simulink model "Perfect_Lineaer"  (R2017a)
settings: Solver=VariableStepAuto  StartTime=0.0  StopTime=17  FixedStep=0.01  RelTol=1e-3
values from neighbouring files (symbols this model uses):
  A = [-4.65E-06	0.0001701	-0.0002836	0	0	0	-2.56E-06	-7.97E-06	3.61E-06 ... (first row only)    [surfaces_setup_test.m]
  A0 = [-4.65E-06	0.0001701	-0.0002836	0	0	0	0	-1.43	0 ... (first row only)    [surfaces_setup_test.m]
  a0_s2345 = [0;0;0.05;0.05]    [HW5_4_surfaces.m]    (also in TEST_aerosetup.m; surfaces_setup_test.m)
  A_2345 = c_2345.*b_2345    [HW5_4_surfaces.m]    (also in TEST_aerosetup.m; surfaces_setup_test.m)
  Aileron_left = 0    [HW5_4_surfaces.m]    (also in TEST_aerosetup.m; surfaces_setup_test.m)
  Aileron_right = 0    [HW5_4_surfaces.m]    (also in TEST_aerosetup.m; surfaces_setup_test.m)
  B = [-7.98E-09	7.83E-09	1.68E-09	2.75E-10 ... (first row only)    [surfaces_setup_test.m]
  B0 = [-6.2	6.2	0	0.45 ... (first row only)    [surfaces_setup_test.m]
  c_2345 = [0.075;0.08;0.1;0.1]    [HW5_4_surfaces.m]    (also in TEST_aerosetup.m; surfaces_setup_test.m)
  CD0_s2345 = [0.01;0.01;0.01;0.01]    [HW5_4_surfaces.m]    (also in TEST_aerosetup.m; surfaces_setup_test.m)
  CDa_s2345 = [1;1;1;1]    [HW5_4_surfaces.m]    (also in TEST_aerosetup.m; surfaces_setup_test.m)
  CL0_2345 = [0;0; 0.05; 0.05]    [HW5_4_surfaces.m]    (also in TEST_aerosetup.m; surfaces_setup_test.m)
  CLa = 2*pi*(r./(2+r))    [HW5_4_surfaces.m]    (also in TEST_aerosetup.m; surfaces_setup_test.m)
  CM0_s2345 = [0;0;-0.05;-0.05]    [HW5_4_surfaces.m]    (also in TEST_aerosetup.m; surfaces_setup_test.m)
  CMa_s2345 = [0; 0; 0; 0]    [HW5_4_surfaces.m]    (also in TEST_aerosetup.m; surfaces_setup_test.m)
  e_s2345 = [0.8;0.8;0.9;0.9]    [HW5_4_surfaces.m]    (also in TEST_aerosetup.m; surfaces_setup_test.m)
  elevator = 0    [HW5_4_surfaces.m]    (also in TEST_aerosetup.m; surfaces_setup_test.m)
  Fext_N = -g_EN * m    [HW5_4_surfaces.m]    (also in TEST_aerosetup.m = [10 10 10]; surfaces_setup_test.m)
  g_EN = [0; 0; 9.81]    [HW5_4_surfaces.m]    (also in TEST_aerosetup.m = [0; 0; 9.8]; surfaces_setup_test.m)
  i_s2345 = [0; 0; 0.05; 0.05;]    [HW5_4_surfaces.m]    (also in TEST_aerosetup.m; surfaces_setup_test.m)
  J_cgp = ones(3)    [surfaces_setup_test.m]
  M_total = sum(MnG(:,1))/1000    [HW5_4_surfaces.m]    (also in TEST_aerosetup.m; surfaces_setup_test.m = sum(MnG1(:,1))/1000)
  Mext_B = [0; 0; 0]    [HW5_4_surfaces.m]    (also in TEST_aerosetup.m = [1; 1; 1]; surfaces_setup_test.m)
  p_E_BE_ini = p_E_BE_ini_deg .* [deg2rad; deg2rad; 1]    [HW5_4_surfaces.m]    (also in TEST_aerosetup.m; surfaces_setup_test.m)
  r = b_2345./c_2345    [HW5_4_surfaces.m]    (also in TEST_aerosetup.m; surfaces_setup_test.m)
  Rearth = 6371000    [HW5_4_surfaces.m]    (also in TEST_aerosetup.m; surfaces_setup_test.m)
  rudder = 0    [HW5_4_surfaces.m]    (also in TEST_aerosetup.m; surfaces_setup_test.m)
  Theta_ini = Theta_ini_deg * deg2rad    [HW5_4_surfaces.m]    (also in TEST_aerosetup.m; surfaces_setup_test.m)
  U0 = [Aileron_right;Aileron_left;elevator;rudder]    [surfaces_setup_test.m]
  v_N_AE = [0;0;0]    [HW5_4_surfaces.m]    (also in TEST_aerosetup.m; surfaces_setup_test.m)
  Vbbe_int = [10; 0; 0]    [HW5_4_surfaces.m]    (also in TEST_aerosetup.m; surfaces_setup_test.m = [5; 0; 0])
  w_B_BE_ini = [1e0; 1e-2; 1e-2]    [HW5_4_surfaces.m]    (also in TEST_aerosetup.m; surfaces_setup_test.m)
  X0 = [w_B_BE_ini;Theta_ini;Vbbe_int]    [surfaces_setup_test.m]
  xyz_s = [[-0.76 0 0.16];[-0.76 0 -0.09];[-0.23 0.44 0];[-0.23 -0.44 0];]    [HW5_4_surfaces.m]    (also in TEST_aerosetup.m; surfaces_setup_test.m)
undefined symbols (not defined in the file or in its folder): Discrete, Earth, K, Time, WGS84
libraries: simulink x83, aerolibfltsims x5, dspsrcs4 x4, simulink_extras x4, dspinverses x3, vrlib x2, sharedtransform x1, aerolibtransform2 x1, aerolibutil x1, sharedutil x1, ctrlSharedLib x1
(part 6 of 8)

== system Perfect_Lineaer/Skid to turn (Lateral Dynamics)1/Subsystem3 ==
  note: Inner loop
  note: State loop
  Rudder : Inport
  A : Gain  Gain=A  Multiplication=Matrix(K*u)
  B : Gain  Gain=B  Multiplication=Matrix(K*u)
  Constant1 : Constant  Value=0
  Constant2 : Constant  Value=X0
  Demux : Demux  Outputs=9
  Integrator : Integrator  InitialConditionSource=external
  KD_Based on Rlocus : Gain
  Mux : Mux  Inputs=9
  Mux1 : Mux
  Scope : Scope
  Scope1 : Scope
  Sum : Sum  Inputs=|++
  Sum1 : Sum  Inputs=|++
  Sum4 : Sum  Inputs=|+-
  selector : Subsystem
  R(yaw) : Outport
  wires:
  Demux/7 -> Mux/7
  Demux/6 -> Mux/6
  Constant2/1 -> Integrator/2
  Demux/3 -> Mux/3
  Sum/1 -> Integrator/1
  selector/1(Out1) -> Scope1/1, KD_Based on Rlocus/1
  B/1 -> Demux/1
  Demux/2 -> Mux/2
  Demux/4 -> Mux/4
  Demux/9 -> Mux/9
  Integrator/1 -> selector/1(In1), Sum4/2, Scope/1, A/1
  Sum4/1 -> Sum/1
  A/1 -> Sum/2
  Demux/5 -> Mux/5
  Demux/1 -> Mux/1
  Mux/1 -> Sum4/1
  Mux1/1 -> B/1
  Constant1/1 -> Mux1/3, Mux1/2, Mux1/1
  Rudder/1 -> Mux1/4
  selector/2(Out2) -> R(yaw)/1
  Demux/8 -> Sum1/1
  KD_Based on Rlocus/1 -> Sum1/2
  Sum1/1 -> Mux/8

== system Perfect_Lineaer/Skid to turn (Lateral Dynamics)1/Subsystem4 ==
  note: Inner loop
  note: State loop
  Rudder : Inport
  A : Gain  Gain=A  Multiplication=Matrix(K*u)
  B : Gain  Gain=B  Multiplication=Matrix(K*u)
  Constant1 : Constant  Value=0
  Constant2 : Constant  Value=X0
  Demux : Demux  Outputs=9
  Integrator : Integrator  InitialConditionSource=external
  KD_Based on Rlocus : Gain
  Mux : Mux  Inputs=9
  Mux1 : Mux
  Scope : Scope
  Scope1 : Scope
  Sum : Sum  Inputs=|++
  Sum1 : Sum  Inputs=|++
  Sum4 : Sum  Inputs=|+-
  selector : Subsystem
  R(yaw) : Outport
  wires:
  Demux/7 -> Mux/7
  Demux/6 -> Mux/6
  Constant2/1 -> Integrator/2
  Demux/3 -> Mux/3
  Sum/1 -> Integrator/1
  selector/1(Out1) -> Scope1/1, KD_Based on Rlocus/1
  B/1 -> Demux/1
  Demux/2 -> Mux/2
  Demux/4 -> Mux/4
  Demux/9 -> Mux/9
  Integrator/1 -> selector/1(In1), Sum4/2, Scope/1, A/1
  Sum4/1 -> Sum/1
  A/1 -> Sum/2
  Demux/5 -> Mux/5
  Demux/1 -> Mux/1
  Mux/1 -> Sum4/1
  Mux1/1 -> B/1
  Constant1/1 -> Mux1/3, Mux1/2, Mux1/1
  Rudder/1 -> Mux1/4
  selector/2(Out2) -> R(yaw)/1
  Demux/8 -> Sum1/1
  KD_Based on Rlocus/1 -> Sum1/2
  Sum1/1 -> Mux/8

== system Perfect_Lineaer/Skid to turn (Lateral Dynamics)1/Subsystem5 ==
  note: Inner loop
  note: State loop
  Rudder : Inport
  Elevator : Inport  Port=2
  A : Gain  Gain=A  Multiplication=Matrix(K*u)
  B : Gain  Gain=B  Multiplication=Matrix(K*u)
  Constant1 : Constant  Value=0
  Constant2 : Constant  Value=X0
  Demux : Demux  Outputs=9
  Integrator : Integrator  InitialConditionSource=external
  KD_Based on Rlocus : Gain
  Mux : Mux  Inputs=9
  Mux1 : Mux
  Scope : Scope
  Scope1 : Scope
  Sum : Sum  Inputs=|++
  Sum1 : Sum  Inputs=|++
  Sum4 : Sum  Inputs=|+-
  selector : Subsystem
  R(yaw) : Outport
  Q(pitch) : Outport  Port=2
  wires:
  Demux/7 -> Mux/7
  Demux/6 -> Mux/6
  Constant2/1 -> Integrator/2
  Demux/3 -> Mux/3
  Sum/1 -> Integrator/1
  selector/1(Out1) -> Scope1/1, KD_Based on Rlocus/1
  B/1 -> Demux/1
  Demux/2 -> Mux/2
  Demux/4 -> Mux/4
  Demux/9 -> Mux/9
  Integrator/1 -> selector/1(In1), Sum4/2, Scope/1, A/1
  Sum4/1 -> Sum/1
  A/1 -> Sum/2
  Demux/5 -> Mux/5
  Demux/1 -> Mux/1
  Mux/1 -> Sum4/1
  Mux1/1 -> B/1
  Constant1/1 -> Mux1/2, Mux1/1
  Rudder/1 -> Mux1/4
  selector/2(yaw) -> R(yaw)/1
  Demux/8 -> Sum1/1
  KD_Based on Rlocus/1 -> Sum1/2
  Sum1/1 -> Mux/8
  selector/3(pitch) -> Q(pitch)/1
  Elevator/1 -> Mux1/3

== system Perfect_Lineaer/Skid to turn (Lateral Dynamics)1/Subsystem6 ==
  note: Inner loop
  note: State loop
  Rudder : Inport
  A : Gain  Gain=A  Multiplication=Matrix(K*u)
  B : Gain  Gain=B  Multiplication=Matrix(K*u)
  Constant1 : Constant  Value=0
  Constant2 : Constant  Value=X0
  Demux : Demux  Outputs=9
  Integrator : Integrator  InitialConditionSource=external
  KD_Based on Rlocus : Gain
  Mux : Mux  Inputs=9
  Mux1 : Mux
  Scope : Scope
  Scope1 : Scope
  Sum : Sum  Inputs=|++
  Sum1 : Sum  Inputs=|++
  Sum4 : Sum  Inputs=|+-
  selector : Subsystem
  R(yaw) : Outport
  wires:
  Demux/7 -> Mux/7
  Demux/6 -> Mux/6
  Constant2/1 -> Integrator/2
  Demux/3 -> Mux/3
  Sum/1 -> Integrator/1
  selector/1(Out1) -> Scope1/1, KD_Based on Rlocus/1
  B/1 -> Demux/1
  Demux/2 -> Mux/2
  Demux/4 -> Mux/4
  Demux/9 -> Mux/9
  Integrator/1 -> selector/1(In1), Sum4/2, Scope/1, A/1
  Sum4/1 -> Sum/1
  A/1 -> Sum/2
  Demux/5 -> Mux/5
  Demux/1 -> Mux/1
  Mux/1 -> Sum4/1
  Mux1/1 -> B/1
  Constant1/1 -> Mux1/3, Mux1/2, Mux1/1
  Rudder/1 -> Mux1/4
  selector/2(Out2) -> R(yaw)/1
  Demux/8 -> Sum1/1
  KD_Based on Rlocus/1 -> Sum1/2
  Sum1/1 -> Mux/8

== system Perfect_Lineaer/Skid to turn (Lateral Dynamics)1/Subsystem7 ==
  note: Inner loop
  note: State loop
  Aileron_r : Inport
  Aileron_l : Inport  Port=2
  A : Gain  Gain=A  Multiplication=Matrix(K*u)
  B : Gain  Gain=B  Multiplication=Matrix(K*u)
  Constant1 : Constant  Value=0
  Constant2 : Constant  Value=X0
  Demux : Demux  Outputs=9
  Integrator : Integrator  InitialConditionSource=external
  KD_Based on Rlocus : Gain
  Mux : Mux  Inputs=9
  Mux1 : Mux
  Scope : Scope
  Scope1 : Scope
  Sum : Sum  Inputs=|++
  Sum1 : Sum  Inputs=|++
  Sum4 : Sum  Inputs=|+-
  selector : Subsystem
  P(roll) : Outport
  wires:
  Demux/7 -> Mux/7
  Demux/6 -> Mux/6
  Constant2/1 -> Integrator/2
  Demux/3 -> Mux/3
  Sum/1 -> Integrator/1
  selector/1(Out1) -> Scope1/1, KD_Based on Rlocus/1
  B/1 -> Demux/1
  Demux/2 -> Mux/2
  Demux/4 -> Mux/4
  Demux/9 -> Mux/9
  Integrator/1 -> selector/1(In1), Sum4/2, Scope/1, A/1
  Sum4/1 -> Sum/1
  A/1 -> Sum/2
  Demux/5 -> Mux/5
  Demux/1 -> Mux/1
  Mux/1 -> Sum4/1
  Mux1/1 -> B/1
  Constant1/1 -> Mux1/3, Mux1/4
  selector/2(Out2) -> P(roll)/1
  Demux/8 -> Sum1/1
  KD_Based on Rlocus/1 -> Sum1/2
  Sum1/1 -> Mux/8
  Aileron_r/1 -> Mux1/1
  Aileron_l/1 -> Mux1/2

== system Perfect_Lineaer/Skid to turn (Lateral Dynamics)1/Subsystem8 ==
  note: Inner loop
  note: State loop
  Aileron_r : Inport
  Aileron_l : Inport  Port=2
  A : Gain  Gain=A  Multiplication=Matrix(K*u)
  B : Gain  Gain=B  Multiplication=Matrix(K*u)
  Constant1 : Constant  Value=0
  Constant2 : Constant  Value=X0
  Demux : Demux  Outputs=9
  Integrator : Integrator  InitialConditionSource=external
  KD_Based on Rlocus : Gain
  Mux : Mux  Inputs=9
  Mux1 : Mux
  Scope : Scope
  Scope1 : Scope
  Sum : Sum  Inputs=|++
  Sum1 : Sum  Inputs=|++
  Sum4 : Sum  Inputs=|+-
  selector : Subsystem
  P(roll) : Outport
  wires:
  Demux/7 -> Mux/7
  Demux/6 -> Mux/6
  Constant2/1 -> Integrator/2
  Demux/3 -> Mux/3
  Sum/1 -> Integrator/1
  selector/1(Out1) -> Scope1/1, KD_Based on Rlocus/1
  B/1 -> Demux/1
  Demux/2 -> Mux/2
  Demux/4 -> Mux/4
  Demux/9 -> Mux/9
  Integrator/1 -> selector/1(In1), Sum4/2, Scope/1, A/1
  Sum4/1 -> Sum/1
  A/1 -> Sum/2
  Demux/5 -> Mux/5
  Demux/1 -> Mux/1
  Mux/1 -> Sum4/1
  Mux1/1 -> B/1
  Constant1/1 -> Mux1/3, Mux1/4
  selector/2(Out2) -> P(roll)/1
  Demux/8 -> Sum1/1
  KD_Based on Rlocus/1 -> Sum1/2
  Sum1/1 -> Mux/8
  Aileron_r/1 -> Mux1/1
  Aileron_l/1 -> Mux1/2

== system Perfect_Lineaer/Skid to turn (Lateral Dynamics)1/Subsystem9 ==
  note: Inner loop
  note: State loop
  Aileron_r : Inport
  Aileron_l : Inport  Port=2
  A : Gain  Gain=A  Multiplication=Matrix(K*u)
  B : Gain  Gain=B  Multiplication=Matrix(K*u)
  Constant1 : Constant  Value=0
  Constant2 : Constant  Value=X0
  Demux : Demux  Outputs=9
  Integrator : Integrator  InitialConditionSource=external
  KD_Based on Rlocus : Gain
  Mux : Mux  Inputs=9
  Mux1 : Mux
  Scope : Scope
  Scope1 : Scope
  Sum : Sum  Inputs=|++
  Sum1 : Sum  Inputs=|++
  Sum4 : Sum  Inputs=|+-
  selector : Subsystem
  P(roll) : Outport
  wires:
  Demux/7 -> Mux/7
  Demux/6 -> Mux/6
  Constant2/1 -> Integrator/2
  Demux/3 -> Mux/3
  Sum/1 -> Integrator/1
  selector/1(Out1) -> Scope1/1, KD_Based on Rlocus/1
  B/1 -> Demux/1
  Demux/2 -> Mux/2
  Demux/4 -> Mux/4
  Demux/9 -> Mux/9
  Integrator/1 -> selector/1(In1), Sum4/2, Scope/1, A/1
  Sum4/1 -> Sum/1
  A/1 -> Sum/2
  Demux/5 -> Mux/5
  Demux/1 -> Mux/1
  Mux/1 -> Sum4/1
  Mux1/1 -> B/1
  Constant1/1 -> Mux1/3, Mux1/4
  selector/2(Out2) -> P(roll)/1
  Demux/8 -> Sum1/1
  KD_Based on Rlocus/1 -> Sum1/2
  Sum1/1 -> Mux/8
  Aileron_l/1 -> Mux1/2
  Aileron_r/1 -> Mux1/1

== system Perfect_Lineaer/Skid to turn (Lateral Dynamics)2/Subsystem ==
  note: State loop
  note: Inner loop
  Rudder : Inport
  A : Gain  Gain=A  Multiplication=Matrix(K*u)
  B : Gain  Gain=B  Multiplication=Matrix(K*u)
  Constant1 : Constant  Value=0
  Constant2 : Constant  Value=X0
  Demux : Demux  Outputs=9
  Integrator : Integrator  InitialConditionSource=external
  KD_Based on Rlocus : Gain
  Mux : Mux  Inputs=9
  Mux1 : Mux
  Scope : Scope
  Scope1 : Scope
  Sum : Sum  Inputs=|++
  Sum1 : Sum  Inputs=|++
  Sum4 : Sum  Inputs=|+-
  selector : Subsystem
  R(yaw) : Outport
  wires:
  Sum1/1 -> Mux/8
  KD_Based on Rlocus/1 -> Sum1/2
  Demux/8 -> Sum1/1
  selector/2(Out2) -> R(yaw)/1
  Rudder/1 -> Mux1/4
  Constant1/1 -> Mux1/1, Mux1/2, Mux1/3
  Mux1/1 -> B/1
  Mux/1 -> Sum4/1
  Demux/1 -> Mux/1
  Demux/5 -> Mux/5
  A/1 -> Sum/2
  Sum4/1 -> Sum/1
  Integrator/1 -> A/1, selector/1(In1), Scope/1, Sum4/2
  Demux/9 -> Mux/9
  Demux/4 -> Mux/4
  Demux/2 -> Mux/2
  B/1 -> Demux/1
  selector/1(Out1) -> KD_Based on Rlocus/1, Scope1/1
  Sum/1 -> Integrator/1
  Demux/3 -> Mux/3
  Constant2/1 -> Integrator/2
  Demux/6 -> Mux/6
  Demux/7 -> Mux/7

== system Perfect_Lineaer/Skid to turn (Lateral Dynamics)2/Subsystem1 ==
  note: State loop
  note: Inner loop
  Elevator : Inport
  A : Gain  Gain=A  Multiplication=Matrix(K*u)
  B : Gain  Gain=B  Multiplication=Matrix(K*u)
  Constant1 : Constant  Value=0
  Constant2 : Constant  Value=X0
  Demux : Demux  Outputs=9
  Integrator : Integrator  InitialConditionSource=external
  KD_Based on Rlocus : Gain
  Mux : Mux  Inputs=9
  Mux1 : Mux
  Scope : Scope
  Scope1 : Scope
  Sum : Sum  Inputs=|++
  Sum1 : Sum  Inputs=|++
  Sum4 : Sum  Inputs=|+-
  selector : Subsystem
  Q(pitch) : Outport
  wires:
  Elevator/1 -> Mux1/3
  Sum1/1 -> Mux/8
  KD_Based on Rlocus/1 -> Sum1/2
  Demux/8 -> Sum1/1
  Constant1/1 -> Mux1/4, Mux1/1, Mux1/2
  Mux1/1 -> B/1
  Mux/1 -> Sum4/1
  Demux/1 -> Mux/1
  Demux/5 -> Mux/5
  A/1 -> Sum/2
  Sum4/1 -> Sum/1
  Integrator/1 -> A/1, Scope/1, Sum4/2, selector/1(In1)
  Demux/9 -> Mux/9
  Demux/4 -> Mux/4
  Demux/2 -> Mux/2
  B/1 -> Demux/1
  selector/1(Out1) -> KD_Based on Rlocus/1, Scope1/1
  Sum/1 -> Integrator/1
  Demux/3 -> Mux/3
  Constant2/1 -> Integrator/2
  Demux/6 -> Mux/6
  Demux/7 -> Mux/7
  selector/2(Out2) -> Q(pitch)/1

== system Perfect_Lineaer/Skid to turn (Lateral Dynamics)2/Subsystem2 ==
  note: State loop
  note: Inner loop
  Rudder : Inport
  A : Gain  Gain=A  Multiplication=Matrix(K*u)
  B : Gain  Gain=B  Multiplication=Matrix(K*u)
  Constant1 : Constant  Value=0
  Constant2 : Constant  Value=X0
  Demux : Demux  Outputs=9
  Integrator : Integrator  InitialConditionSource=external
  KD_Based on Rlocus : Gain
  Mux : Mux  Inputs=9
  Mux1 : Mux
  Scope : Scope
  Scope1 : Scope
  Sum : Sum  Inputs=|++
  Sum1 : Sum  Inputs=|++
  Sum4 : Sum  Inputs=|+-
  selector : Subsystem
  R(yaw) : Outport
  wires:
  Sum1/1 -> Mux/8
  KD_Based on Rlocus/1 -> Sum1/2
  Demux/8 -> Sum1/1
  selector/2(Out2) -> R(yaw)/1
  Rudder/1 -> Mux1/4
  Constant1/1 -> Mux1/1, Mux1/2, Mux1/3
  Mux1/1 -> B/1
  Mux/1 -> Sum4/1
  Demux/1 -> Mux/1
  Demux/5 -> Mux/5
  A/1 -> Sum/2
  Sum4/1 -> Sum/1
  Integrator/1 -> A/1, Scope/1, Sum4/2, selector/1(In1)
  Demux/9 -> Mux/9
  Demux/4 -> Mux/4
  Demux/2 -> Mux/2
  B/1 -> Demux/1
  selector/1(Out1) -> KD_Based on Rlocus/1, Scope1/1
  Sum/1 -> Integrator/1
  Demux/3 -> Mux/3
  Constant2/1 -> Integrator/2
  Demux/6 -> Mux/6
  Demux/7 -> Mux/7

== system Perfect_Lineaer/Skid to turn (Lateral Dynamics)2/Subsystem3 ==
  note: State loop
  note: Inner loop
  Elevator : Inport
  A : Gain  Gain=A  Multiplication=Matrix(K*u)
  B : Gain  Gain=B  Multiplication=Matrix(K*u)
  Constant1 : Constant  Value=0
  Constant2 : Constant  Value=X0
  Demux : Demux  Outputs=9
  Integrator : Integrator  InitialConditionSource=external
  KD_Based on Rlocus : Gain
  Mux : Mux  Inputs=9
  Mux1 : Mux
  Scope : Scope
  Scope1 : Scope
  Sum : Sum  Inputs=|++
  Sum1 : Sum  Inputs=|++
  Sum4 : Sum  Inputs=|+-
  selector : Subsystem
  Q(pitch) : Outport
  wires:
  Elevator/1 -> Mux1/3
  Sum1/1 -> Mux/8
  KD_Based on Rlocus/1 -> Sum1/2
  Demux/8 -> Sum1/1
  Constant1/1 -> Mux1/4, Mux1/1, Mux1/2
  Mux1/1 -> B/1
  Mux/1 -> Sum4/1
  Demux/1 -> Mux/1
  Demux/5 -> Mux/5
  A/1 -> Sum/2
  Sum4/1 -> Sum/1
  Integrator/1 -> A/1, Scope/1, Sum4/2, selector/1(In1)
  Demux/9 -> Mux/9
  Demux/4 -> Mux/4
  Demux/2 -> Mux/2
  B/1 -> Demux/1
  selector/1(Out1) -> KD_Based on Rlocus/1, Scope1/1
  Sum/1 -> Integrator/1
  Demux/3 -> Mux/3
  Constant2/1 -> Integrator/2
  Demux/6 -> Mux/6
  Demux/7 -> Mux/7
  selector/2(Out2) -> Q(pitch)/1

== system Perfect_Lineaer/Skid to turn (Lateral Dynamics)2/Subsystem4 ==
  note: State loop
  note: Inner loop
  Elevator : Inport
  A : Gain  Gain=A  Multiplication=Matrix(K*u)
  B : Gain  Gain=B  Multiplication=Matrix(K*u)
  Constant1 : Constant  Value=0
  Constant2 : Constant  Value=X0
  Demux : Demux  Outputs=9
  Integrator : Integrator  InitialConditionSource=external
  KD_Based on Rlocus : Gain
  Mux : Mux  Inputs=9
  Mux1 : Mux
  Scope : Scope
  Scope1 : Scope
  Sum : Sum  Inputs=|++
  Sum1 : Sum  Inputs=|++
  Sum4 : Sum  Inputs=|+-
  selector : Subsystem
  Theta : Outport
  wires:
  Elevator/1 -> Mux1/3
  Sum1/1 -> Mux/8
  KD_Based on Rlocus/1 -> Sum1/2
  Demux/8 -> Sum1/1
  Constant1/1 -> Mux1/4, Mux1/1, Mux1/2
  Mux1/1 -> B/1
  Mux/1 -> Sum4/1
  Demux/1 -> Mux/1
  Demux/5 -> Mux/5
  A/1 -> Sum/2
  Sum4/1 -> Sum/1
  Integrator/1 -> A/1, Scope/1, Sum4/2, selector/1(In1)
  Demux/9 -> Mux/9
  Demux/4 -> Mux/4
  Demux/2 -> Mux/2
  B/1 -> Demux/1
  selector/1(Out1) -> KD_Based on Rlocus/1, Scope1/1
  Sum/1 -> Integrator/1
  Demux/3 -> Mux/3
  Constant2/1 -> Integrator/2
  Demux/6 -> Mux/6
  Demux/7 -> Mux/7
  selector/2(Out2) -> Theta/1

== system Perfect_Lineaer/Skid to turn (Lateral Dynamics)2/Subsystem5 ==
  note: State loop
  note: Inner loop
  Rudder : Inport
  Elevator : Inport  Port=2
  A : Gain  Gain=A  Multiplication=Matrix(K*u)
  B : Gain  Gain=B  Multiplication=Matrix(K*u)
  Constant1 : Constant  Value=0
  Constant2 : Constant  Value=X0
  Demux : Demux  Outputs=9
  Integrator : Integrator  InitialConditionSource=external
  KD_Based on Rlocus : Gain
  Mux : Mux  Inputs=9
  Mux1 : Mux
  Scope : Scope
  Scope1 : Scope
  Sum : Sum  Inputs=|++
  Sum1 : Sum  Inputs=|++
  Sum4 : Sum  Inputs=|+-
  selector : Subsystem
  R(yaw) : Outport
  Q(pitch) : Outport  Port=2
  wires:
  Elevator/1 -> Mux1/3
  Sum1/1 -> Mux/8
  KD_Based on Rlocus/1 -> Sum1/2
  Demux/8 -> Sum1/1
  Rudder/1 -> Mux1/4
  Constant1/1 -> Mux1/1, Mux1/2
  Mux1/1 -> B/1
  Mux/1 -> Sum4/1
  Demux/1 -> Mux/1
  Demux/5 -> Mux/5
  A/1 -> Sum/2
  Sum4/1 -> Sum/1
  Integrator/1 -> A/1, selector/1(In1), Scope/1, Sum4/2
  Demux/9 -> Mux/9
  Demux/4 -> Mux/4
  Demux/2 -> Mux/2
  B/1 -> Demux/1
  selector/1(Out1) -> KD_Based on Rlocus/1, Scope1/1
  Sum/1 -> Integrator/1
  Demux/3 -> Mux/3
  Constant2/1 -> Integrator/2
  Demux/6 -> Mux/6
  Demux/7 -> Mux/7
  selector/2(Out2) -> Q(pitch)/1
  selector/3(Out3) -> R(yaw)/1

== system Perfect_Lineaer/Skid to turn (Lateral Dynamics)2/Subsystem6 ==
  note: State loop
  note: Inner loop
  Rudder : Inport
  A : Gain  Gain=A  Multiplication=Matrix(K*u)
  B : Gain  Gain=B  Multiplication=Matrix(K*u)
  Constant1 : Constant  Value=0
  Constant2 : Constant  Value=X0
  Demux : Demux  Outputs=9
  Integrator : Integrator  InitialConditionSource=external
  KD_Based on Rlocus : Gain
  Mux : Mux  Inputs=9
  Mux1 : Mux
  Scope : Scope
  Scope1 : Scope
  Sum : Sum  Inputs=|++
  Sum1 : Sum  Inputs=|++
  Sum4 : Sum  Inputs=|+-
  selector : Subsystem
  R(yaw) : Outport
  wires:
  Sum1/1 -> Mux/8
  KD_Based on Rlocus/1 -> Sum1/2
  Demux/8 -> Sum1/1
  selector/2(Out2) -> R(yaw)/1
  Rudder/1 -> Mux1/4
  Constant1/1 -> Mux1/1, Mux1/2, Mux1/3
  Mux1/1 -> B/1
  Mux/1 -> Sum4/1
  Demux/1 -> Mux/1
  Demux/5 -> Mux/5
  A/1 -> Sum/2
  Sum4/1 -> Sum/1
  Integrator/1 -> A/1, Scope/1, Sum4/2, selector/1(In1)
  Demux/9 -> Mux/9
  Demux/4 -> Mux/4
  Demux/2 -> Mux/2
  B/1 -> Demux/1
  selector/1(Out1) -> KD_Based on Rlocus/1, Scope1/1
  Sum/1 -> Integrator/1
  Demux/3 -> Mux/3
  Constant2/1 -> Integrator/2
  Demux/6 -> Mux/6
  Demux/7 -> Mux/7

== system Perfect_Lineaer/Skid to turn (Lateral Dynamics)2/Subsystem7 ==
  note: State loop
  note: Inner loop
  Aileron_r : Inport
  Aileron_l : Inport  Port=2
  A : Gain  Gain=A  Multiplication=Matrix(K*u)
  B : Gain  Gain=B  Multiplication=Matrix(K*u)
  Constant1 : Constant  Value=0
  Constant2 : Constant  Value=X0
  Demux : Demux  Outputs=9
  Integrator : Integrator  InitialConditionSource=external
  KD_Based on Rlocus : Gain
  Mux : Mux  Inputs=9
  Mux1 : Mux
  Scope : Scope
  Scope1 : Scope
  Sum : Sum  Inputs=|++
  Sum1 : Sum  Inputs=|++
  Sum4 : Sum  Inputs=|+-
  selector : Subsystem
  P(roll) : Outport
  wires:
  Aileron_l/1 -> Mux1/2
  Aileron_r/1 -> Mux1/1
  Sum1/1 -> Mux/8
  KD_Based on Rlocus/1 -> Sum1/2
  Demux/8 -> Sum1/1
  selector/2(Out2) -> P(roll)/1
  Constant1/1 -> Mux1/4, Mux1/3
  Mux1/1 -> B/1
  Mux/1 -> Sum4/1
  Demux/1 -> Mux/1
  Demux/5 -> Mux/5
  A/1 -> Sum/2
  Sum4/1 -> Sum/1
  Integrator/1 -> A/1, selector/1(In1), Scope/1, Sum4/2
  Demux/9 -> Mux/9
  Demux/4 -> Mux/4
  Demux/2 -> Mux/2
  B/1 -> Demux/1
  selector/1(Out1) -> KD_Based on Rlocus/1, Scope1/1
  Sum/1 -> Integrator/1
  Demux/3 -> Mux/3
  Constant2/1 -> Integrator/2
  Demux/6 -> Mux/6
  Demux/7 -> Mux/7

== system Perfect_Lineaer/Skid to turn (Lateral Dynamics)2/Subsystem8 ==
  note: State loop
  note: Inner loop
  Aileron_r : Inport
  Aileron_l : Inport  Port=2
  A : Gain  Gain=A  Multiplication=Matrix(K*u)
  B : Gain  Gain=B  Multiplication=Matrix(K*u)
  Constant1 : Constant  Value=0
  Constant2 : Constant  Value=X0
  Demux : Demux  Outputs=9
  Integrator : Integrator  InitialConditionSource=external
  KD_Based on Rlocus : Gain
  Mux : Mux  Inputs=9
  Mux1 : Mux
  Scope : Scope
  Scope1 : Scope
  Sum : Sum  Inputs=|++
  Sum1 : Sum  Inputs=|++
  Sum4 : Sum  Inputs=|+-
  selector : Subsystem
  P(roll) : Outport
  wires:
  Aileron_l/1 -> Mux1/2
  Aileron_r/1 -> Mux1/1
  Sum1/1 -> Mux/8
  KD_Based on Rlocus/1 -> Sum1/2
  Demux/8 -> Sum1/1
  selector/2(Out2) -> P(roll)/1
  Constant1/1 -> Mux1/4, Mux1/3
  Mux1/1 -> B/1
  Mux/1 -> Sum4/1
  Demux/1 -> Mux/1
  Demux/5 -> Mux/5
  A/1 -> Sum/2
  Sum4/1 -> Sum/1
  Integrator/1 -> A/1, selector/1(In1), Scope/1, Sum4/2
  Demux/9 -> Mux/9
  Demux/4 -> Mux/4
  Demux/2 -> Mux/2
  B/1 -> Demux/1
  selector/1(Out1) -> KD_Based on Rlocus/1, Scope1/1
  Sum/1 -> Integrator/1
  Demux/3 -> Mux/3
  Constant2/1 -> Integrator/2
  Demux/6 -> Mux/6
  Demux/7 -> Mux/7

== system Perfect_Lineaer/Skid to turn (Lateral Dynamics)2/Subsystem9 ==
  note: State loop
  note: Inner loop
  Aileron_r : Inport
  Aileron_l : Inport  Port=2
  A : Gain  Gain=A  Multiplication=Matrix(K*u)
  B : Gain  Gain=B  Multiplication=Matrix(K*u)
  Constant1 : Constant  Value=0
  Constant2 : Constant  Value=X0
  Demux : Demux  Outputs=9
  Integrator : Integrator  InitialConditionSource=external
  KD_Based on Rlocus : Gain
  Mux : Mux  Inputs=9
  Mux1 : Mux
  Scope : Scope
  Scope1 : Scope
  Sum : Sum  Inputs=|++
  Sum1 : Sum  Inputs=|++
  Sum4 : Sum  Inputs=|+-
  selector : Subsystem
  P(roll) : Outport
  wires:
  Aileron_r/1 -> Mux1/1
  Aileron_l/1 -> Mux1/2
  Sum1/1 -> Mux/8
  KD_Based on Rlocus/1 -> Sum1/2
  Demux/8 -> Sum1/1
  selector/2(Out2) -> P(roll)/1
  Constant1/1 -> Mux1/4, Mux1/3
  Mux1/1 -> B/1
  Mux/1 -> Sum4/1
  Demux/1 -> Mux/1
  Demux/5 -> Mux/5
  A/1 -> Sum/2
  Sum4/1 -> Sum/1
  Integrator/1 -> A/1, selector/1(In1), Scope/1, Sum4/2
  Demux/9 -> Mux/9
  Demux/4 -> Mux/4
  Demux/2 -> Mux/2
  B/1 -> Demux/1
  selector/1(Out1) -> KD_Based on Rlocus/1, Scope1/1
  Sum/1 -> Integrator/1
  Demux/3 -> Mux/3
  Constant2/1 -> Integrator/2
  Demux/6 -> Mux/6
  Demux/7 -> Mux/7

== system Perfect_Lineaer/Subsystem1/Subsystem ==
  note: Inner loop
  note: State loop
  Rudder : Inport
  A : Gain  Gain=A  Multiplication=Matrix(K*u)
  B : Gain  Gain=B  Multiplication=Matrix(K*u)
  Constant1 : Constant  Value=0
  Constant2 : Constant  Value=X0
  Demux : Demux  Outputs=9
  Integrator : Integrator  InitialConditionSource=external
  KD_Based on Rlocus : Gain
  Mux : Mux  Inputs=9
  Mux1 : Mux
  Scope : Scope
  Scope1 : Scope
  Sum : Sum  Inputs=|++
  Sum1 : Sum  Inputs=|++
  Sum4 : Sum  Inputs=|+-
  selector : Subsystem
  R(yaw) : Outport
  wires:
  Demux/7 -> Mux/7
  Demux/6 -> Mux/6
  Constant2/1 -> Integrator/2
  Demux/3 -> Mux/3
  Sum/1 -> Integrator/1
  selector/1(Out1) -> Scope1/1, KD_Based on Rlocus/1
  B/1 -> Demux/1
  Demux/2 -> Mux/2
  Demux/4 -> Mux/4
  Demux/9 -> Mux/9
  Integrator/1 -> selector/1(In1), Sum4/2, Scope/1, A/1
  Sum4/1 -> Sum/1
  A/1 -> Sum/2
  Demux/5 -> Mux/5
  Demux/1 -> Mux/1
  Mux/1 -> Sum4/1
  Mux1/1 -> B/1
  Constant1/1 -> Mux1/3, Mux1/2, Mux1/1
  Rudder/1 -> Mux1/4
  selector/2(Out2) -> R(yaw)/1
  Demux/8 -> Sum1/1
  KD_Based on Rlocus/1 -> Sum1/2
  Sum1/1 -> Mux/8

== system Perfect_Lineaer/Subsystem1/Subsystem1 ==
  note: Inner loop
  note: State loop
  Elevator : Inport
  A : Gain  Gain=A  Multiplication=Matrix(K*u)
  B : Gain  Gain=B  Multiplication=Matrix(K*u)
  Constant1 : Constant  Value=0
  Constant2 : Constant  Value=X0
  Demux : Demux  Outputs=9
  Integrator : Integrator  InitialConditionSource=external
  KD_Based on Rlocus : Gain
  Mux : Mux  Inputs=9
  Mux1 : Mux
  Scope : Scope
  Scope1 : Scope
  Sum : Sum  Inputs=|++
  Sum1 : Sum  Inputs=|++
  Sum4 : Sum  Inputs=|+-
  selector : Subsystem
  Q(pitch) : Outport
  wires:
  Demux/7 -> Mux/7
  Demux/6 -> Mux/6
  Constant2/1 -> Integrator/2
  Demux/3 -> Mux/3
  Sum/1 -> Integrator/1
  selector/1(Out1) -> Scope1/1, KD_Based on Rlocus/1
  B/1 -> Demux/1
  Demux/2 -> Mux/2
  Demux/4 -> Mux/4
  Demux/9 -> Mux/9
  Integrator/1 -> selector/1(In1), Sum4/2, Scope/1, A/1
  Sum4/1 -> Sum/1
  A/1 -> Sum/2
  Demux/5 -> Mux/5
  Demux/1 -> Mux/1
  Mux/1 -> Sum4/1
  Mux1/1 -> B/1
  Constant1/1 -> Mux1/2, Mux1/1, Mux1/4
  selector/2(Out2) -> Q(pitch)/1
  Demux/8 -> Sum1/1
  KD_Based on Rlocus/1 -> Sum1/2
  Sum1/1 -> Mux/8
  Elevator/1 -> Mux1/3

== system Perfect_Lineaer/Subsystem1/Subsystem5 ==
  note: Inner loop
  note: State loop
  Rudder : Inport
  Elevator : Inport  Port=2
  A : Gain  Gain=A  Multiplication=Matrix(K*u)
  B : Gain  Gain=B  Multiplication=Matrix(K*u)
  Constant1 : Constant  Value=0
  Constant2 : Constant  Value=X0
  Demux : Demux  Outputs=9
  Integrator : Integrator  InitialConditionSource=external
  KD_Based on Rlocus : Gain
  Mux : Mux  Inputs=9
  Mux1 : Mux
  Scope : Scope
  Scope1 : Scope
  Sum : Sum  Inputs=|++
  Sum1 : Sum  Inputs=|++
  Sum4 : Sum  Inputs=|+-
  selector : Subsystem
  R(yaw) : Outport
  Q(pitch) : Outport  Port=2
  wires:
  Demux/7 -> Mux/7
  Demux/6 -> Mux/6
  Constant2/1 -> Integrator/2
  Demux/3 -> Mux/3
  Sum/1 -> Integrator/1
  selector/1(Out1) -> Scope1/1, KD_Based on Rlocus/1
  B/1 -> Demux/1
  Demux/2 -> Mux/2
  Demux/4 -> Mux/4
  Demux/9 -> Mux/9
  Integrator/1 -> selector/1(In1), Sum4/2, Scope/1, A/1
  Sum4/1 -> Sum/1
  A/1 -> Sum/2
  Demux/5 -> Mux/5
  Demux/1 -> Mux/1
  Mux/1 -> Sum4/1
  Mux1/1 -> B/1
  Constant1/1 -> Mux1/2, Mux1/1
  Rudder/1 -> Mux1/4
  selector/2(yaw) -> R(yaw)/1
  Demux/8 -> Sum1/1
  KD_Based on Rlocus/1 -> Sum1/2
  Sum1/1 -> Mux/8
  selector/3(pitch) -> Q(pitch)/1
  Elevator/1 -> Mux1/3

== system Perfect_Lineaer/Washout/Subsystem ==
  note: State loop
  note: Inner loop
  Rudder : Inport
  A : Gain  Gain=A  Multiplication=Matrix(K*u)
  B : Gain  Gain=B  Multiplication=Matrix(K*u)
  Constant1 : Constant  Value=0
  Constant2 : Constant  Value=X0
  Demux : Demux  Outputs=9
  Integrator : Integrator  InitialConditionSource=external
  KD_Based on Rlocus : Gain
  Mux : Mux  Inputs=9
  Mux1 : Mux
  Scope : Scope
  Scope1 : Scope
  Sum : Sum  Inputs=|++
  Sum1 : Sum  Inputs=|++
  Sum4 : Sum  Inputs=|+-
  selector : Subsystem
  R(yaw) : Outport
  wires:
  Sum1/1 -> Mux/8
  KD_Based on Rlocus/1 -> Sum1/2
  Demux/8 -> Sum1/1
  selector/2(Out2) -> R(yaw)/1
  Rudder/1 -> Mux1/4
  Constant1/1 -> Mux1/1, Mux1/2, Mux1/3
  Mux1/1 -> B/1
  Mux/1 -> Sum4/1
  Demux/1 -> Mux/1
  Demux/5 -> Mux/5
  A/1 -> Sum/2
  Sum4/1 -> Sum/1
  Integrator/1 -> A/1, selector/1(In1), Scope/1, Sum4/2
  Demux/9 -> Mux/9
  Demux/4 -> Mux/4
  Demux/2 -> Mux/2
  B/1 -> Demux/1
  selector/1(Out1) -> KD_Based on Rlocus/1, Scope1/1
  Sum/1 -> Integrator/1
  Demux/3 -> Mux/3
  Constant2/1 -> Integrator/2
  Demux/6 -> Mux/6
  Demux/7 -> Mux/7

== system Perfect_Lineaer/Washout/Subsystem1 ==
  note: State loop
  note: Inner loop
  Rudder : Inport
  A : Gain  Gain=A  Multiplication=Matrix(K*u)
  B : Gain  Gain=B  Multiplication=Matrix(K*u)
  Constant1 : Constant  Value=0
  Constant2 : Constant  Value=X0
  Demux : Demux  Outputs=9
  Integrator : Integrator  InitialConditionSource=external
  KD_Based on Rlocus : Gain
  Mux : Mux  Inputs=9
  Mux1 : Mux
  Scope : Scope
  Scope1 : Scope
  Sum : Sum  Inputs=|++
  Sum1 : Sum  Inputs=|++
  Sum4 : Sum  Inputs=|+-
  selector : Subsystem
  R(yaw) : Outport
  Psi : Outport  Port=2
  wires:
  Sum1/1 -> Mux/8
  KD_Based on Rlocus/1 -> Sum1/2
  Demux/8 -> Sum1/1
  selector/2(Out2) -> R(yaw)/1
  Rudder/1 -> Mux1/4
  Constant1/1 -> Mux1/1, Mux1/2, Mux1/3
  Mux1/1 -> B/1
  Mux/1 -> Sum4/1
  Demux/1 -> Mux/1
  Demux/5 -> Mux/5
  A/1 -> Sum/2
  Sum4/1 -> Sum/1
  Integrator/1 -> A/1, selector/1(In1), Scope/1, Sum4/2
  Demux/9 -> Mux/9
  Demux/4 -> Mux/4
  Demux/2 -> Mux/2
  B/1 -> Demux/1
  selector/1(Out1) -> KD_Based on Rlocus/1, Scope1/1
  Sum/1 -> Integrator/1
  Demux/3 -> Mux/3
  Constant2/1 -> Integrator/2
  Demux/6 -> Mux/6
  Demux/7 -> Mux/7
  selector/3(Out3) -> Psi/1

== system Perfect_Lineaer/Washout/Subsystem2 ==
  note: Inner loop
  note: State loop
  Rudder : Inport
  A : Gain  Gain=A  Multiplication=Matrix(K*u)
  "A_l, A_r &Elevator" : Constant  Value=0
  B : Gain  Gain=B  Multiplication=Matrix(K*u)
  Constant2 : Constant  Value=X0
  Demux : Demux  Outputs=9
  Integrator : Integrator  InitialConditionSource=external
  KD : Gain
  Mux : Mux  Inputs=9
  Mux1 : Mux
  Sum : Sum  Inputs=|++
  Sum1 : Sum  Inputs=|++
  Sum4 : Sum  Inputs=|+-
  selector : Subsystem
  R(yaw) : Outport
  wires:
  Demux/7 -> Mux/7
  Demux/6 -> Mux/6
  Constant2/1 -> Integrator/2
  Demux/3 -> Mux/3
  Sum/1 -> Integrator/1
  selector/1(Out1) -> KD/1
  B/1 -> Demux/1
  Demux/2 -> Mux/2
  Demux/4 -> Mux/4
  Demux/9 -> Mux/9
  Integrator/1 -> selector/1(In1), Sum4/2, A/1
  Sum4/1 -> Sum/1
  A/1 -> Sum/2
  Demux/5 -> Mux/5
  Demux/1 -> Mux/1
  Mux/1 -> Sum4/1
  Mux1/1 -> B/1
  "A_l, A_r &Elevator"/1 -> Mux1/3, Mux1/2, Mux1/1
  Rudder/1 -> Mux1/4
  selector/2(Out2) -> R(yaw)/1
  Demux/8 -> Sum1/1
  KD/1 -> Sum1/2
  Sum1/1 -> Mux/8

== system Perfect_Lineaer/Washout/Subsystem3 ==
  note: Inner loop
  note: State loop
  Rudder : Inport
  A : Gain  Gain=A  Multiplication=Matrix(K*u)
  B : Gain  Gain=B  Multiplication=Matrix(K*u)
  Constant1 : Constant  Value=0
  Constant2 : Constant  Value=X0
  Demux : Demux  Outputs=9
  Integrator : Integrator  InitialConditionSource=external
  KD_Based on Rlocus : Gain
  Mux : Mux  Inputs=9
  Mux1 : Mux
  Scope : Scope
  Scope1 : Scope
  Sum : Sum  Inputs=|++
  Sum1 : Sum  Inputs=|++
  Sum4 : Sum  Inputs=|+-
  selector : Subsystem
  R(yaw) : Outport
  wires:
  Demux/7 -> Mux/7
  Demux/6 -> Mux/6
  Constant2/1 -> Integrator/2
  Demux/3 -> Mux/3
  Sum/1 -> Integrator/1
  selector/1(Out1) -> Scope1/1, KD_Based on Rlocus/1
  B/1 -> Demux/1
  Demux/2 -> Mux/2
  Demux/4 -> Mux/4
  Demux/9 -> Mux/9
  Integrator/1 -> selector/1(In1), Sum4/2, Scope/1, A/1
  Sum4/1 -> Sum/1
  A/1 -> Sum/2
  Demux/5 -> Mux/5
  Demux/1 -> Mux/1
  Mux/1 -> Sum4/1
  Mux1/1 -> B/1
  Constant1/1 -> Mux1/3, Mux1/2, Mux1/1
  Rudder/1 -> Mux1/4
  selector/2(Out2) -> R(yaw)/1
  Demux/8 -> Sum1/1
  KD_Based on Rlocus/1 -> Sum1/2
  Sum1/1 -> Mux/8

== system Perfect_Lineaer/Washout/Subsystem4 ==
  note: Inner loop
  note: State loop
  Rudder : Inport
  A : Gain  Gain=A  Multiplication=Matrix(K*u)
  B : Gain  Gain=B  Multiplication=Matrix(K*u)
  Constant1 : Constant  Value=0
  Constant2 : Constant  Value=X0
  Demux : Demux  Outputs=9
  Integrator : Integrator  InitialConditionSource=external
  KD_Based on Rlocus : Gain
  Mux : Mux  Inputs=9
  Mux1 : Mux
  Scope : Scope
  Scope1 : Scope
  Sum : Sum  Inputs=|++
  Sum1 : Sum  Inputs=|++
  Sum4 : Sum  Inputs=|+-
  selector : Subsystem
  R(yaw) : Outport
  wires:
  Demux/7 -> Mux/7
  Demux/6 -> Mux/6
  Constant2/1 -> Integrator/2
  Demux/3 -> Mux/3
  Sum/1 -> Integrator/1
  selector/1(Out1) -> Scope1/1, KD_Based on Rlocus/1
  B/1 -> Demux/1
  Demux/2 -> Mux/2
  Demux/4 -> Mux/4
  Demux/9 -> Mux/9
  Integrator/1 -> selector/1(In1), Sum4/2, Scope/1, A/1
  Sum4/1 -> Sum/1
  A/1 -> Sum/2
  Demux/5 -> Mux/5
  Demux/1 -> Mux/1
  Mux/1 -> Sum4/1
  Mux1/1 -> B/1
  Constant1/1 -> Mux1/3, Mux1/2, Mux1/1
  Rudder/1 -> Mux1/4
  selector/2(Out2) -> R(yaw)/1
  Demux/8 -> Sum1/1
  KD_Based on Rlocus/1 -> Sum1/2
  Sum1/1 -> Mux/8

== system Perfect_Lineaer/with surf1_PID/selector ==
  note: Outer loop
  In1 : Inport
  Demux : Demux  Outputs=9
  Gain : Gain  Gain=pi/180
  Mux : Mux  Inputs=9
  Mux1 : Mux  Inputs=3
  Terminator : Terminator
  Phi : Outport
  Out2 : Outport  Port=2
  V : Outport  Port=3
  wires:
  In1/1 -> Demux/1
  Mux/1 -> Terminator/1
  Mux1/1 -> Gain/1
  Gain/1 -> Out2/1
  Demux/1 -> Mux/1
  Demux/2 -> Mux/2
  Demux/3 -> Mux/3
  Demux/4 -> Mux1/1, Phi/1, Mux/4
  Demux/5 -> Mux1/2, Mux/5
  Demux/6 -> Mux1/3, Mux/6
  Demux/7 -> Mux/7
  Demux/8 -> V/1, Mux/8
  Demux/9 -> Mux/9

== system Perfect_Lineaer/All together/Subsystem1/AeroSurface controller ==
  V_inf : Inport
  Alp : Inport  Port=2
  Beta : Inport  Port=3
  V_B_BA : Inport  Port=4
  ar : Inport  Port=5
  al : Inport  Port=6
  e : Inport  Port=7
  r : Inport  Port=8
  Complex to Real-Imag : ComplexToRealImag
  Complex to Real-Imag1 : ComplexToRealImag
  Gain : Gain  Gain=1/1000
  Gain1 : Gain  Gain=1/1000
  MATLAB Function : MATLAB Function  TreatAsAtomicUnit=on
  Terminator : Terminator
  Terminator1 : Terminator
  F : Outport
  M : Outport  Port=2
  wires:
  V_inf/1 -> MATLAB Function/2(V_inf)
  V_B_BA/1 -> MATLAB Function/1(V_B_BA)
  ar/1 -> MATLAB Function/5(aileron_r)
  al/1 -> MATLAB Function/6(aileron_l)
  e/1 -> MATLAB Function/7(elevator)
  r/1 -> MATLAB Function/8(rudder)
  Alp/1 -> MATLAB Function/3(alp)
  Beta/1 -> MATLAB Function/4(bet)
  MATLAB Function/1(F_b) -> Complex to Real-Imag/1
  Complex to Real-Imag/1 -> Gain/1
  Complex to Real-Imag/2 -> Terminator/1
  MATLAB Function/2(M_b) -> Complex to Real-Imag1/1
  Complex to Real-Imag1/2 -> Terminator1/1
  Complex to Real-Imag1/1 -> Gain1/1
  Gain/1 -> F/1
  Gain1/1 -> M/1

== system Perfect_Lineaer/All together/Subsystem1/Airspeed Indicator ==

== system Perfect_Lineaer/All together/Subsystem1/Altimeter ==

== system Perfect_Lineaer/All together/Subsystem1/Artificial Horizon ==

== system Perfect_Lineaer/All together/Subsystem1/Climb Rate Indicator ==

== system Perfect_Lineaer/All together/Subsystem1/Rot dyn1 ==
  Mext_B : Inport
  J_cg : Inport  Port=2
  ini_rates : Inport  Port=3
  " LU Inverse" : dspinverses/ LU Inverse
      settings: SourceProductName=DSP System Toolbox
  Add : Sum  Inputs=+-
  Cross Product : vrlib/Utilities/Cross Product
      settings: SourceProductBaseCode=VR
  Integrator : Integrator  InitialConditionSource=external
  Matrix Multiply : Product  Multiplication=Matrix(*)
  Matrix Multiply1 : Product  Multiplication=Matrix(*)
  om_B_B_BE : Outport
  wires:
  Matrix Multiply/1 -> Cross Product/2
  Add/1 -> Matrix Multiply1/2
  Cross Product/1 -> Add/2
  Matrix Multiply1/1 -> Integrator/1
  ini_rates/1 -> Integrator/2
  Integrator/1 -> Cross Product/1, Matrix Multiply/2, om_B_B_BE/1
  Mext_B/1 -> Add/1
  J_cg/1 -> Matrix Multiply/1, " LU Inverse"/1
  " LU Inverse"/1 -> Matrix Multiply1/1

== system Perfect_Lineaer/All together/Subsystem1/Rot kine ==
  om_B_B_BE : Inport
  Theta_ini : Inport  Port=2
  ROLL desire : Inport  Port=3
  ROLL desire1 : Inport  Port=4
  Constant : Constant  Value=0
  Demux : Demux  Commented=on  Outputs=3
  Demux1 : Demux  Outputs=3
  "Euler to Quat " : MATLAB Function  TreatAsAtomicUnit=on
  Euler to Quat 1 : MATLAB Function  TreatAsAtomicUnit=on
  Euler to Quat 3 : MATLAB Function  TreatAsAtomicUnit=on
  Gain : Gain  Gain=1/2
  Integrator : Integrator  InitialConditionSource=external
  Integrator1 : Integrator  InitialConditionSource=external
  Integrator2 : Integrator  InitialConditionSource=external
  Matrix Multiply : Product  Multiplication=Matrix(*)
  Matrix Multiply1 : Product  Multiplication=Matrix(*)
  Mux : Mux  Inputs=2
  Mux1 : Mux  Commented=on  Inputs=3
  Mux2 : Mux  Inputs=4'
  PID Controller : simulink/Continuous/PID Controller  Commented=on  Controller=PID  TimeDomain=Continuous-time  SampleTime=-1  IntegratorMethod=Forward Euler  FilterMethod=Forward Euler  Form=Parallel  UseFilter=on  ControllerParametersSource=internal  P=0  I=10  D=0  N=100  InitialConditionSource=internal  InitialConditionForIntegrator=0  InitialConditionForFilter=0  ExternalReset=none  LimitOutput=off  UpperSaturationLimit=inf  LowerSaturationLimit=-inf  LinearizeAsGain=on  AntiWindupMode=none  Kb=1  TrackingMode=off  Kt=1  PParamMin=[]  PParamMax=[]  IParamMin=[]  IParamMax=[]  DParamMin=[]  DParamMax=[]  NParamMin=[]  NParamMax=[]  KbParamMin=[]  KbParamMax=[]  KtParamMin=[]  KtParamMax=[]  POutMin=[]  POutMax=[]  IOutMin=[]  IOutMax=[]  DOutMin=[]  DOutMax=[]  NOutMin=[]  NOutMax=[]  KbOutMin=[]  KbOutMax=[]  KtOutMin=[]  KtOutMax=[]  IntegratorOutMin=[]  IntegratorOutMax=[]  FilterOutMin=[]  FilterOutMax=[]  SumOutMin=[]  SumOutMax=[]  SumI1OutMin=[]  SumI1OutMax=[]  SumI2OutMin=[]  SumI2OutMax=[]  SumI3OutMin=[]  SumI3OutMax=[]  SumDOutMin=[]  SumDOutMax=[]  SaturationOutMin=[]  SaturationOutMax=[]  IntegratorContinuousStateAttributes=''  IntegratorStateMustResolveToSignalObject=off  IntegratorRTWStateStorageClass=Auto  FilterContinuousStateAttributes=''  FilterStateMustResolveToSignalObject=off  FilterRTWStateStorageClass=Auto  DifferentiatorICPrevScaledInput=0  DifferentiatorOutMin=[]  DifferentiatorOutMax=[]  InitialConditionSetting=State (most efficient)
  PID Controller1 : simulink/Continuous/PID Controller  Controller=PID  TimeDomain=Continuous-time  SampleTime=-1  IntegratorMethod=Forward Euler  FilterMethod=Forward Euler  Form=Parallel  UseFilter=on  ControllerParametersSource=internal  P=0  I=-1  D=0  N=100  InitialConditionSource=internal  InitialConditionForIntegrator=0  InitialConditionForFilter=0  ExternalReset=none  LimitOutput=off  UpperSaturationLimit=inf  LowerSaturationLimit=-inf  LinearizeAsGain=on  AntiWindupMode=none  Kb=1  TrackingMode=off  Kt=1  PParamMin=[]  PParamMax=[]  IParamMin=[]  IParamMax=[]  DParamMin=[]  DParamMax=[]  NParamMin=[]  NParamMax=[]  KbParamMin=[]  KbParamMax=[]  KtParamMin=[]  KtParamMax=[]  POutMin=[]  POutMax=[]  IOutMin=[]  IOutMax=[]  DOutMin=[]  DOutMax=[]  NOutMin=[]  NOutMax=[]  KbOutMin=[]  KbOutMax=[]  KtOutMin=[]  KtOutMax=[]  IntegratorOutMin=[]  IntegratorOutMax=[]  FilterOutMin=[]  FilterOutMax=[]  SumOutMin=[]  SumOutMax=[]  SumI1OutMin=[]  SumI1OutMax=[]  SumI2OutMin=[]  SumI2OutMax=[]  SumI3OutMin=[]  SumI3OutMax=[]  SumDOutMin=[]  SumDOutMax=[]  SaturationOutMin=[]  SaturationOutMax=[]  IntegratorContinuousStateAttributes=''  IntegratorStateMustResolveToSignalObject=off  IntegratorRTWStateStorageClass=Auto  FilterContinuousStateAttributes=''  FilterStateMustResolveToSignalObject=off  FilterRTWStateStorageClass=Auto  DifferentiatorICPrevScaledInput=0  DifferentiatorOutMin=[]  DifferentiatorOutMax=[]  InitialConditionSetting=State (most efficient)
  Quat2Euler 1 : MATLAB Function  TreatAsAtomicUnit=on
  Quaternion Division : aerolibutil/Quaternion Division
      settings: SourceProductName=Aerospace Blockset  SourceProductBaseCode=AE
  Quaternion Normalize : sharedutil/Quaternion Normalize
  Scope : Scope
  Scope1 : Scope  Commented=on
  Scope2 : Scope  Commented=on
  Scope3 : Scope
  Sum : Sum  Commented=on  Inputs=|++
  Sum1 : Sum  Commented=on  Inputs=|+-
  Sum2 : Sum  Inputs=|+-
  Sum3 : Sum  Inputs=|++
  ATT_1 : Outport
  ATT_quat : Outport  Port=2
  wires:
  om_B_B_BE/1 -> Demux1/1, Matrix Multiply1/2, Matrix Multiply/2
  Integrator/1 -> Sum3/2, Sum2/2, Scope/1, ATT_1/1, Demux/1
  "Euler to Quat "/1(H) -> Matrix Multiply/1
  Theta_ini/1 -> Euler to Quat 3/1(att), Integrator/2, Integrator1/2  "Theta_ini"
  Matrix Multiply/1 -> Integrator/1
  Demux/3 -> Sum/2, Mux/2
  Demux/1 -> Mux1/1
  PID Controller/1 -> Sum1/2, Mux/1, Mux1/3
  Mux/1 -> Scope1/1
  Demux/2 -> Mux1/2
  Mux1/1 -> Scope2/1
  ROLL desire/1 -> Sum1/1
  Sum1/1 -> Sum/1
  Sum/1 -> PID Controller/1
  Sum2/1 -> PID Controller1/1
  ROLL desire1/1 -> Sum2/1
  PID Controller1/1 -> Sum3/1
  Sum3/1 -> "Euler to Quat "/1(att)
  Integrator1/1 -> Euler to Quat 1/1(att), Scope3/1
  Matrix Multiply1/1 -> Integrator1/1
  Euler to Quat 1/1(H) -> Matrix Multiply1/1
  Quaternion Normalize/1 -> Quat2Euler 1/1(Q), Quaternion Division/1
  Demux1/3 -> Mux2/4
  Integrator2/1 -> Quaternion Normalize/1
  Demux1/1 -> Mux2/2
  Quaternion Division/1 -> Gain/1
  Constant/1 -> Mux2/1
  Gain/1 -> Integrator2/1
  Mux2/1 -> Quaternion Division/2
  Demux1/2 -> Mux2/3
  Quat2Euler 1/1(theta) -> ATT_quat/1
  Euler to Quat 3/1(Q) -> Integrator2/2

== system Perfect_Lineaer/All together/Subsystem1/Subsystem ==
  In1 : Inport
  Demux : Demux  Outputs=3
  Gain : Gain  Gain=180/pi
  Mux : Mux  Inputs=2
  Terminator : Terminator
  Out1 : Outport
  wires:
  In1/1 -> Gain/1
  Demux/2 -> Mux/1
  Demux/3 -> Mux/2
  Mux/1 -> Out1/1
  Demux/1 -> Terminator/1
  Gain/1 -> Demux/1

== system Perfect_Lineaer/All together/Subsystem1/Subsystem1 ==
  In1 : Inport
  Out1 : Outport
  wires:
  In1/1 -> Out1/1

== system Perfect_Lineaer/All together/Subsystem1/Trans Dyn1 ==
  Fext_B : Inport
  g_B : Inport  Port=2
  om_B_B_BE : Inport  Port=3
  m : Inport  Port=4
  V_initi : Inport  Port=5
  Add : Sum  Inputs=++-
  Cross Product : vrlib/Utilities/Cross Product
      settings: SourceProductBaseCode=VR
  Divide : Product  Inputs=*/
  Integrator : Integrator  InitialConditionSource=external
  Xdot_E_B_BE : Outport
  wires:
  Fext_B/1 -> Divide/1
  m/1 -> Divide/2
  Divide/1 -> Add/1
  g_B/1 -> Add/2
  om_B_B_BE/1 -> Cross Product/1
  Cross Product/1 -> Add/3
  Add/1 -> Integrator/1
  V_initi/1 -> Integrator/2
  Integrator/1 -> Cross Product/2, Xdot_E_B_BE/1

== system Perfect_Lineaer/All together/Subsystem1/atmosphere ==
  C_BN : Inport
  v_N_AE(wind NED) : Inport  Port=2
  Matrix Multiply : Product  Multiplication=Matrix(*)
  v_B_AE : Outport
  wires:
  v_N_AE(wind NED)/1 -> Matrix Multiply/2
  C_BN/1 -> Matrix Multiply/1
  Matrix Multiply/1 -> v_B_AE/1

== system Perfect_Lineaer/All together/Subsystem1/new tran kine sph ==
  V_E_B_BE : Inport
  C_NB : Inport  Port=2
  Rearth : Inport  Port=3
  p_BE_E_ini : Inport  Port=4
  " LU Inverse" : dspinverses/ LU Inverse
      settings: SourceProductName=DSP System Toolbox
  C_EB : Product  Multiplication=Matrix(*)
  Integrator : Integrator  InitialConditionSource=external
  Scope : Scope
  V_EB1 : Product  Multiplication=Matrix(*)
  X_EE 2 P_EE : Subsystem
  X_EE 2 P_EE1 : Subsystem
  p2Cne : Subsystem
  sph_trans : MATLAB Function  TreatAsAtomicUnit=on
  X_E_E-BE : Outport
  p_e_e_be1 : Outport  Port=2
  Xdot_E_E-BE1 : Outport  Port=3
  wires:
  " LU Inverse"/1 -> C_EB/1
  Integrator/1 -> Scope/1, X_E_E-BE/1, X_EE 2 P_EE/1(X_E_E_BE), X_EE 2 P_EE1/1(X_E_E_BE)
  X_EE 2 P_EE1/1(P_E_E_BE) -> p_e_e_be1/1
  Rearth/1 -> X_EE 2 P_EE1/2(Rearth), X_EE 2 P_EE/2(Rearth)
  V_EB1/1 -> Xdot_E_E-BE1/1, Integrator/1
  C_EB/1 -> V_EB1/1
  p2Cne/1(C-NE) -> " LU Inverse"/1
  X_EE 2 P_EE/1(P_E_E_BE) -> p2Cne/1(p_E_E_BE)
  C_NB/1 -> C_EB/2
  V_E_B_BE/1 -> V_EB1/2
  p_BE_E_ini/1 -> sph_trans/1(P_BE_E_ini)
  sph_trans/1(X_BE_E_ini) -> Integrator/2

== system Perfect_Lineaer/All together/Subsystem1/wind axes vector ==
  v_B_BA(vx vy vz) : Inport
  Atan2 : Trigonometry  Operator=atan2
  Constant : Constant  Value=0.001
  Constant1 : Constant  Value=[0,0,0]
  Demux : Demux  Outputs=3
  Divide : Product  Inputs=*/
  Dot Product : DotProduct  InputSameDT=on  OutDataTypeStr=Inherit: Inherit via internal rule
  MinMax : MinMax  Function=max  Inputs=2
  Mux : Mux  Inputs=3
  Saturation : Saturate
  Sqrt : Sqrt  SaturateOnIntegerOverflow=on
  Switch : Switch  Criteria=u2 > Threshold
  Trigonometric Function : Trigonometry  Operator=asin  ApproximationMethod=CORDIC
  w_B_BA : Outport
  wires:
  v_B_BA(vx vy vz)/1 -> Demux/1, Dot Product/2, Dot Product/1
  Dot Product/1 -> Sqrt/1
  Sqrt/1 -> Mux/1, Switch/2, MinMax/1
  Constant/1 -> MinMax/2
  MinMax/1 -> Divide/2
  Demux/2 -> Divide/1
  Demux/3 -> Atan2/1
  Demux/1 -> Atan2/2
  Atan2/1 -> Mux/2
  Divide/1 -> Saturation/1
  Saturation/1 -> Trigonometric Function/1
  Trigonometric Function/1 -> Mux/3
  Constant1/1 -> Switch/3
  Mux/1 -> Switch/1
  Switch/1 -> w_B_BA/1

== system Perfect_Lineaer/All together/Subsystem2/selector ==
  note: Outer loop
  In1 : Inport
  Demux : Demux  Outputs=9
  Demux1 : Demux  Outputs=3
  MATLAB Function : MATLAB Function  TreatAsAtomicUnit=on
  Mux : Mux  Inputs=8
  Mux1 : Mux  Inputs=3
  Scope : Scope
  Terminator : Terminator
  Out1 : Outport
  Out2 : Outport  Port=2
  Out3 : Outport  Port=3
  Out4 : Outport  Port=4
  wires:
  MATLAB Function/1(euler_dot) -> Demux1/1
  Demux1/1 -> Out4/1
  In1/1 -> Demux/1
  Demux/9 -> Mux/8
  Demux/5 -> MATLAB Function/2(theta), Mux/5, Mux1/2
  Demux/2 -> MATLAB Function/5(R), Mux/2
  Demux/6 -> Mux/6, Mux1/3
  Demux/1 -> MATLAB Function/4(Q), MATLAB Function/3(P), Mux/1
  Demux/3 -> Mux/3
  Mux/1 -> Terminator/1
  Demux/7 -> Mux/7
  Demux/4 -> MATLAB Function/1(phi), Mux/4, Mux1/1
  Demux1/2 -> Out2/1
  Demux/8 -> Out1/1
  Mux1/1 -> Scope/1
  Demux1/3 -> Out3/1

== system Perfect_Lineaer/All together/Subsystem5/selector ==
  note: Outer loop
  In1 : Inport
  Demux : Demux  Outputs=9
  Demux1 : Demux  Outputs=3
  MATLAB Function : MATLAB Function  TreatAsAtomicUnit=on
  Mux : Mux  Inputs=8
  Mux1 : Mux  Inputs=3
  Scope : Scope
  Terminator : Terminator
  Out1 : Outport
  Out2 : Outport  Port=2
  Out3 : Outport  Port=3
  Out4 : Outport  Port=4
  wires:
  MATLAB Function/1(euler_dot) -> Demux1/1
  Demux1/1 -> Out4/1
  In1/1 -> Demux/1
  Demux/9 -> Mux/8
  Demux/5 -> MATLAB Function/2(theta), Mux/5, Mux1/2
  Demux/2 -> MATLAB Function/5(R), Mux/2
  Demux/6 -> Mux/6, Mux1/3
  Demux/1 -> MATLAB Function/4(Q), MATLAB Function/3(P), Mux/1
  Demux/3 -> Mux/3
  Mux/1 -> Terminator/1
  Demux/7 -> Mux/7
  Demux/4 -> MATLAB Function/1(phi), Mux/4, Mux1/1
  Demux1/2 -> Out2/1
  Demux/8 -> Out1/1
  Mux1/1 -> Scope/1
  Demux1/3 -> Out3/1

== system Perfect_Lineaer/Command size/Subsystem/selector ==
  note: Outer loop
  In1 : Inport
  Demux : Demux  Outputs=9
  Demux1 : Demux  Outputs=3
  MATLAB Function : MATLAB Function  TreatAsAtomicUnit=on
  Mux : Mux  Inputs=8
  Mux1 : Mux  Inputs=3
  Scope : Scope
  Terminator : Terminator
  Terminator1 : Terminator
  Terminator2 : Terminator
  Out1 : Outport
  Out2 : Outport  Port=2
  wires:
  MATLAB Function/1(euler_dot) -> Demux1/1
  Demux1/1 -> Terminator1/1
  In1/1 -> Demux/1
  Demux/9 -> Mux/8
  Demux/5 -> MATLAB Function/2(theta), Mux/5, Mux1/2
  Demux/2 -> MATLAB Function/5(R), Mux/2
  Demux/6 -> Mux/6, Mux1/3
  Demux/1 -> MATLAB Function/4(Q), MATLAB Function/3(P), Mux/1
  Demux/3 -> Mux/3
  Mux/1 -> Terminator/1
  Demux/7 -> Mux/7
  Demux/4 -> MATLAB Function/1(phi), Mux/4, Mux1/1
  Demux/8 -> Out1/1
  Mux1/1 -> Scope/1
  Demux1/3 -> Out2/1
  Demux1/2 -> Terminator2/1

== system Perfect_Lineaer/Command size/Subsystem1/selector ==
  note: Outer loop
  In1 : Inport
  Demux : Demux  Outputs=9
  Demux1 : Demux  Outputs=3
  MATLAB Function : MATLAB Function  TreatAsAtomicUnit=on
  Mux : Mux  Inputs=8
  Mux1 : Mux  Inputs=3
  Scope : Scope
  Terminator : Terminator
  Terminator1 : Terminator
  Terminator2 : Terminator
  Out1 : Outport
  Out2 : Outport  Port=2
  wires:
  Mux1/1 -> Scope/1
  Demux/9 -> Mux/8
  Demux/8 -> Out1/1
  Mux/1 -> Terminator/1
  Demux/7 -> Mux/7
  Demux/6 -> Mux/6, Mux1/3
  Demux/4 -> MATLAB Function/1(phi), Mux/4, Mux1/1
  In1/1 -> Demux/1
  Demux/2 -> MATLAB Function/5(R), Mux/2
  Demux/3 -> Mux/3
  Demux/1 -> MATLAB Function/4(Q), MATLAB Function/3(P), Mux/1
  Demux/5 -> MATLAB Function/2(theta), Mux/5, Mux1/2
  MATLAB Function/1(euler_dot) -> Demux1/1
  Demux1/2 -> Out2/1
  Demux1/1 -> Terminator1/1
  Demux1/3 -> Terminator2/1

== system Perfect_Lineaer/Command size/Subsystem2/selector ==
  note: Outer loop
  In1 : Inport
  Demux : Demux  Outputs=9
  Demux1 : Demux  Outputs=3
  MATLAB Function : MATLAB Function  TreatAsAtomicUnit=on
  Mux : Mux  Inputs=8
  Mux1 : Mux  Inputs=3
  Scope : Scope
  Terminator : Terminator
  Terminator1 : Terminator
  Terminator2 : Terminator
  Out1 : Outport
  Out2 : Outport  Port=2
  wires:
  MATLAB Function/1(euler_dot) -> Demux1/1
  Demux1/1 -> Terminator1/1
  In1/1 -> Demux/1
  Demux/9 -> Mux/8
  Demux/5 -> MATLAB Function/2(theta), Mux/5, Mux1/2
  Demux/2 -> MATLAB Function/5(R), Mux/2
  Demux/6 -> Mux/6, Mux1/3
  Demux/1 -> MATLAB Function/4(Q), MATLAB Function/3(P), Mux/1
  Demux/3 -> Mux/3
  Mux/1 -> Terminator/1
  Demux/7 -> Mux/7
  Demux/4 -> MATLAB Function/1(phi), Mux/4, Mux1/1
  Demux/8 -> Out1/1
  Mux1/1 -> Scope/1
  Demux1/3 -> Out2/1
  Demux1/2 -> Terminator2/1
